simulink model "Simulink_Linearization_Model"  (R2022b)
settings: Solver=FixedStepAuto  StartTime=0.0  StopTime=200  FixedStep=0.001  RelTol=1e-3
undefined symbols (not defined in the file or in its folder): G, power_rated
libraries: simulink_extras x1, simulink x1
settings Model: Creator=ka402286  LastModifiedBy=mo780715
settings DataIOCC: SaveState=on
settings OptimizationCC: BlockReduction=off  DefaultParameterBehavior=Inlined  BufferReuse=off
settings ModelReferenceCC: EnableRefExpFcnMdlSchedulingChecks=on
settings RTWCC: RetainRTWFile=on  CustomInclude="\"C:\\Users\\ka402286\\Documents\\PhD Reseacrh\\Fatigue Load reduction Using IPC(By Dq and Atlas Theory)\\Linearization\\FMIKit-Simulink-2.9\\include\" \"C:\\Users\\ka402286\\Documents\\PhD Reseacrh\\Fatigue Load reduction Using IPC(By Dq and Atlas Theory)\\Load Reduction\\FMIKit-Simulink-2.9\\include\" \"C:\\Users\\ka402286\\Documents\\test\\FMIKit-Simulink-2.9\\include\" \"C:\\Users\\ka402286\\Documents\\PhD Reseacrh\\Fatigue load reduction based on RGA\\CRAFTS_Model_at_different_azimuth\\FMIKit-Simulink-2.9\\include\""  CustomSource="\"C:\\Users\\ka402286\\Documents\\PhD Reseacrh\\Fatigue Load reduction Using IPC(By Dq and Atlas Theory)\\Linearization\\FMIKit-Simulink-2.9\\src\\FMU.cpp\" \"C:\\Users\\ka402286\\Documents\\PhD Reseacrh\\Fatigue Load reduction Using IPC(By Dq and Atlas Theory)\\Linearization\\FMIKit-Simulink-2.9\\src\\FMU1.cpp\" \"C:\\Users\\ka402286\\Documents\\PhD Reseacrh\\Fatigue Load reduction Using IPC(By Dq and Atlas Theory)\\Linearization\\FMIKit-Simulink-2.9\\src\\FMU2.cpp\" \"C:\\Users\\ka402286\\Documents\\PhD Reseacrh\\Fatigue Load reduction Using IPC(By Dq and Atlas Theory)\\Load Reduction\\FMIKit-Simulink-2.9\\src\\FMU.cpp\" \"C:\\Users\\ka402286\\Documents\\PhD Reseacrh\\Fatigue Load reduction Using IPC(By Dq and Atlas Theory)\\Load Reduction\\FMIKit-Simulink-2.9\\src\\FMU1.cpp\" \"C:\\Users\\ka402286\\Documents\\PhD Reseacrh\\Fatigue Load reduction Using IPC(By Dq and Atlas Theory)\\Load Reduction\\FMIKit-Simulink-2.9\\src\\FMU2.cpp\" \"C:\\Users\\ka402286\\Documents\\test\\FMIKit-Simulink-2.9\\src\\FMU.cpp\" \"C:\\Users\\ka402286\\Documents\\test\\FMIKit-Simulink-2.9\\src\\FMU1.cpp\" \"C:\\Users\\ka402286\\Documents\\test\\FMIKit-Simulink-2.9\\src\\FMU2.cpp\" \"C:\\Users\\ka402286\\Documents\\PhD Reseacrh\\Fatigue load reduction based on RGA\\CRAFTS_Model_at_different_azimuth\\FMIKit-Simulink-2.9\\src\\FMU.cpp\" \"C:\\Users\\ka402286\\Documents\\PhD Reseacrh\\Fatigue load reduction based on RGA\\CRAFTS_Model_at_different_azimuth\\FMIKit-Simulink-2.9\\src\\FMU1.cpp\" \"C:\\Users\\ka402286\\Documents\\PhD Reseacrh\\Fatigue load reduction based on RGA\\CRAFTS_Model_at_different_azimuth\\FMIKit-Simulink-2.9\\src\\FMU2.cpp\""

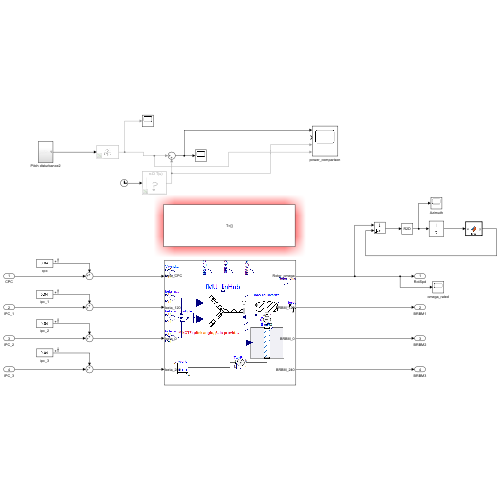
[thumbnail: Simulink's stored preview of the top-level diagram]
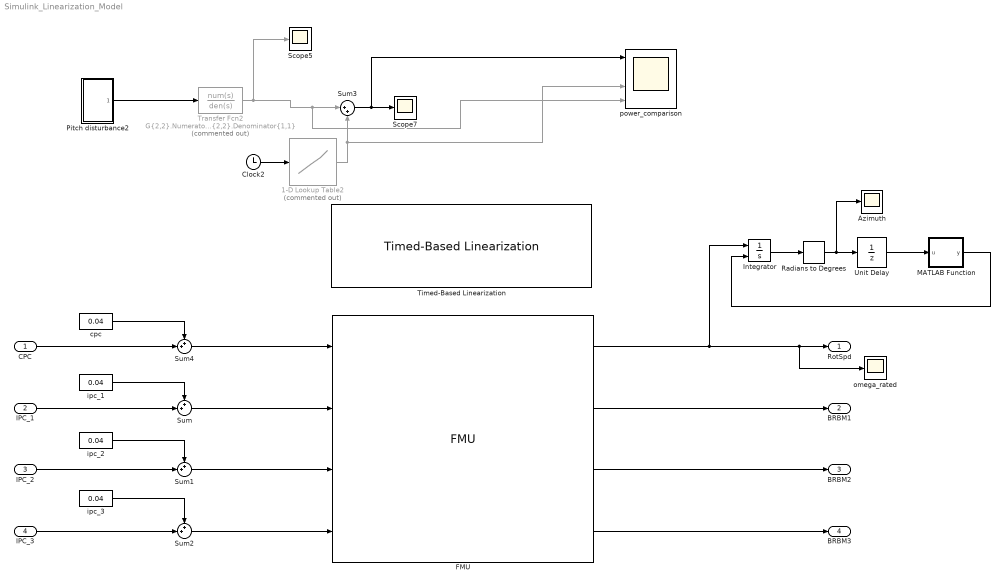
== system Simulink_Linearization_Model ==
  CPC : Inport
  IPC_1 : Inport  Port=2
  IPC_2 : Inport  Port=3
  IPC_3 : Inport  Port=4
  1-D Lookup Table2 : Lookup_n-D  Commented=on  NumberOfTableDimensions=1  BreakpointsForDimension1=power_rated(:,1)  Table=power_rated(:,2)  InternalRulePriority=Speed  RndMeth=Simplest
  Azimuth : Scope
  Clock2 : Clock
  FMU : FMU  FMUName=FMU_QFT_MIMO_Regime3_StaticWind.fmu  FMUMode=ModelExchange
      settings: MultithreadedSim=off
      mask Type: FMU_QFT_MIMO_Regime3_StaticWind [Model Exchange, v2.0]
      mask Display:
      | if (exist([Simulink.fileGenControl('get','CacheFolder') '\slprj\_fmu\584540f2eb884b768e5422b012e8c2aa\FMU_QFT_MIMO_Regime3_StaticWind\model.png'],'file'))
      |     image([Simulink.fileGenControl('get','CacheFolder') '\slprj\_fmu\584540f2eb884b768e5422b012e8c2aa\FMU_QFT_MIMO_Regime3_StaticWind\model.png']);
      | else
      |     disp('FMU_QFT_MIMO_Regime3_StaticWind');
      | end
      | port_label('output',1,'Rotor_omega');
      | port_label('output',2,'BRBM_120');
      | port_label('output',3,'BRBM_0');
      | port_label('output',4,'BRBM_240');
      | port_label('input',1,'beta_CPC');
      | port_label('input',2,'beta_120');
      | port_label('input',3,'beta_0');
      | port_label('input',4,'beta_240');
  Integrator : Integrator  ExternalReset=rising
  MATLAB Function : MATLAB Function  TreatAsAtomicUnit=on
  Pitch disturbance2 : Subsystem
  Radians to Degrees : simulink_extras/Transformations/Radians to Degrees
  Scope5 : Scope
  Scope7 : Scope
  Sum{,1..2,4} (4 alike) : Sum  Inputs=++|
  Sum3 : Sum  Inputs=|++
  Timed-Based Linearization : simulink/Model-Wide Utilities/Timed-Based Linearization  LinearizationTime=t_linearization  SampleTime=0
  Transfer Fcn2 : TransferFcn  Commented=on  Numerator=G{2,2}.Numerator{1,1}  Denominator=G{2,2}.Denominator{1,1}
  Unit Delay : UnitDelay  SampleTime=-1  HasFrameUpgradeWarning=on
  cpc : Constant  Value=0.04
  ipc_1 : Constant  Value=0.04
  ipc_2 : Constant  Value=0.04
  ipc_3 : Constant  Value=0.04
  omega_rated : Scope
  power_comparison : Scope  NumInputPorts=4
  RotSpd : Outport
  BRBM1 : Outport  Port=2
  BRBM2 : Outport  Port=3
  BRBM3 : Outport  Port=4
  wires:
  FMU/2 -> BRBM1/1
  FMU/3 -> BRBM2/1
  FMU/4 -> BRBM3/1
  FMU/1 -> Integrator/1, RotSpd/1, omega_rated/1
  Sum3/1 -> power_comparison/1, Scope7/1
  Pitch disturbance2/1(Output) -> Transfer Fcn2/1
  Transfer Fcn2/1 -> Scope5/1, power_comparison/4, Sum3/1
  Clock2/1 -> 1-D Lookup Table2/1
  1-D Lookup Table2/1 -> power_comparison/3, Sum3/2
  Integrator/1 -> Radians to Degrees/1
  Radians to Degrees/1 -> Azimuth/1, Unit Delay/1
  Unit Delay/1 -> MATLAB Function/1(u)
  MATLAB Function/1(y) -> Integrator/2
  ipc_1/1 -> Sum/1
  IPC_1/1 -> Sum/2
  Sum/1 -> FMU/2
  ipc_2/1 -> Sum1/1
  Sum1/1 -> FMU/3
  IPC_2/1 -> Sum1/2
  ipc_3/1 -> Sum2/1
  Sum2/1 -> FMU/4
  IPC_3/1 -> Sum2/2
  Sum4/1 -> FMU/1
  cpc/1 -> Sum4/1
  CPC/1 -> Sum4/2

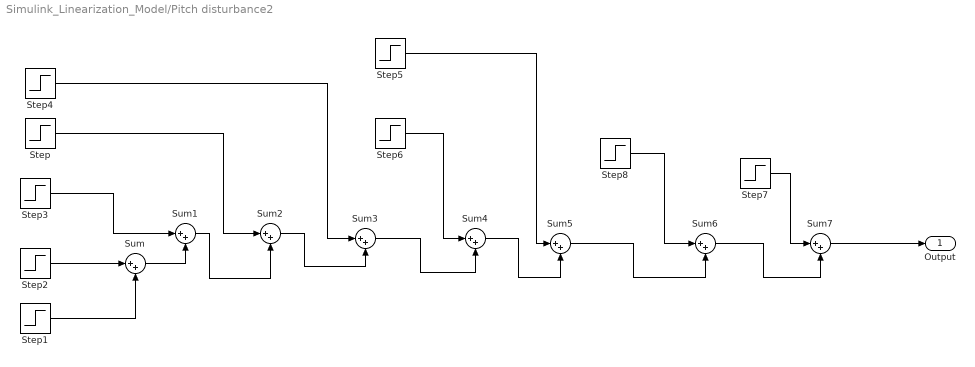
== system Simulink_Linearization_Model/Pitch disturbance2 ==
  Step : Step  Time=150  After=.01  SampleTime=0
  Step1 : Step  After=-.02  SampleTime=0
  Step2 : Step  Time=50  After=.01  SampleTime=0
  Step3 : Step  Time=100  After=.01  SampleTime=0
  Step4 : Step  Time=200  After=.01  SampleTime=0
  Step5 : Step  Time=300  After=-.01  SampleTime=0
  Step6 : Step  Time=250  After=-.01  SampleTime=0
  Step7 : Step  Time=400  After=-.01  SampleTime=0
  Step8 : Step  Time=350  After=-.01  SampleTime=0
  Sum{,1..7} (8 alike) : Sum  Inputs=|++
  Output : Outport
  wires:
  Step1/1 -> Sum/2
  Sum/1 -> Sum1/2
  Step2/1 -> Sum/1
  Sum5/1 -> Sum6/2
  Sum7/1 -> Output/1
  Step4/1 -> Sum3/1
  Sum2/1 -> Sum3/2
  Sum4/1 -> Sum5/2
  Sum6/1 -> Sum7/2
  Step3/1 -> Sum1/1
  Sum3/1 -> Sum4/2
  Step/1 -> Sum2/1
  Sum1/1 -> Sum2/2
  Step6/1 -> Sum4/1
  Step7/1 -> Sum7/1
  Step8/1 -> Sum6/1
  Step5/1 -> Sum5/1

== matlab function Simulink_Linearization_Model/MATLAB Function ==
  data: u input; y output
function y = fcn(u)
    if u >= 360
        y = 1;
    else
        y = 0;
    end
end
